simulink model "sim_pid_genetic"  (R2016b)
settings: Solver=ode5  StartTime=0.0  StopTime=10  FixedStep=0.01  RelTol=1e-3
values from neighbouring files (symbols this model uses):
  kd_ws = kd_val_dec(member,:)    [sim_genetic.m]
  ki_ws = ki_val_dec(member,:)    [sim_genetic.m]
  kp_ws = kp_val_dec(member,:)    [sim_genetic.m]
undefined symbols (not defined in the file or in its folder): DiscIntNeverNeededParam
settings Model: Creator=ismail.uzunlar  LastModifiedBy=Ismail

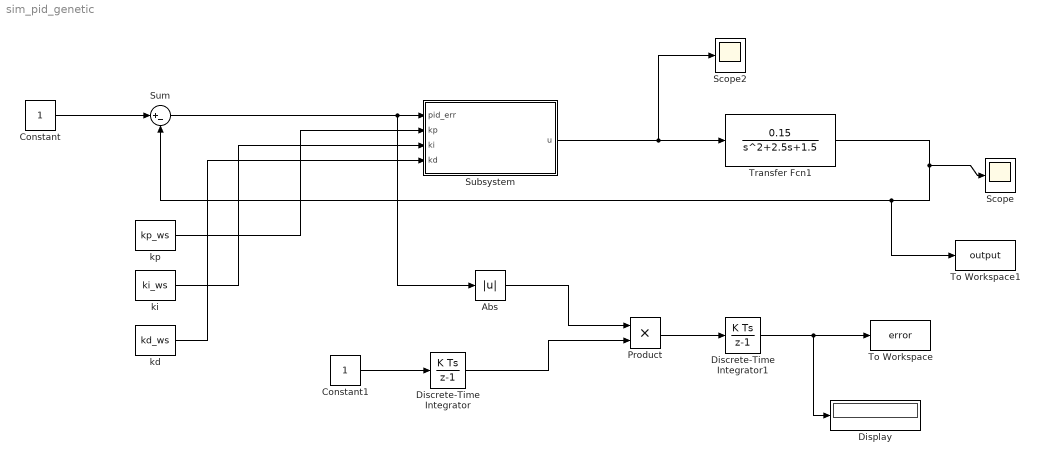
== system sim_pid_genetic ==
  Abs : Abs
  Constant : Constant
  Constant1 : Constant
  Discrete-Time Integrator : DiscreteIntegrator  gainval=1  InitialConditionSetting=State (most efficient)  SampleTime=-1  ICPrevOutput=DiscIntNeverNeededParam  ICPrevScaledInput=DiscIntNeverNeededParam
  Discrete-Time Integrator1 : DiscreteIntegrator  gainval=100  InitialConditionSetting=State (most efficient)  SampleTime=-1  ICPrevOutput=DiscIntNeverNeededParam  ICPrevScaledInput=DiscIntNeverNeededParam
  Display : Display
  Product : Product
  Scope : Scope
  Scope2 : Scope
  Subsystem : Subsystem
  Sum : Sum  Inputs=|+-
  To Workspace : ToWorkspace  VariableName=error  SaveFormat=Timeseries  SampleTime=-1
  To Workspace1 : ToWorkspace  VariableName=output  SaveFormat=Timeseries  SampleTime=-1
  Transfer Fcn1 : TransferFcn  Numerator=[0.15]  Denominator=[1 2.5 1.5]
  kd : Constant  Value=kd_ws
  ki : Constant  Value=ki_ws
  kp : Constant  Value=kp_ws
  wires:
  Subsystem/1(u) -> Scope2/1, Transfer Fcn1/1
  Constant/1 -> Sum/1
  Sum/1 -> Abs/1, Subsystem/1(pid_err)
  Transfer Fcn1/1 -> To Workspace1/1, Sum/2, Scope/1
  kp/1 -> Subsystem/2(kp)
  ki/1 -> Subsystem/3(ki)
  kd/1 -> Subsystem/4(kd)
  Constant1/1 -> Discrete-Time Integrator/1
  Discrete-Time Integrator/1 -> Product/2
  Abs/1 -> Product/1
  Product/1 -> Discrete-Time Integrator1/1
  Discrete-Time Integrator1/1 -> Display/1, To Workspace/1

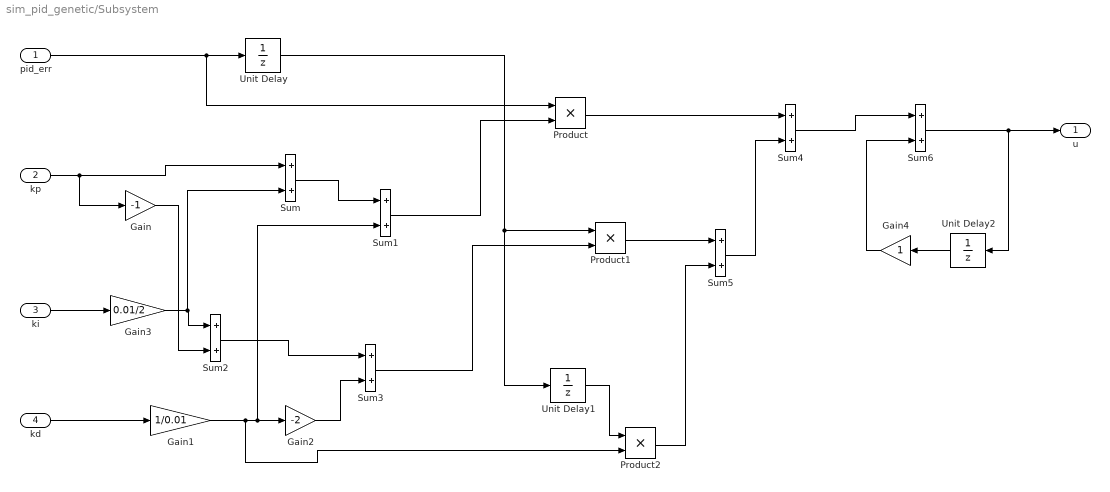
== system sim_pid_genetic/Subsystem ==
  pid_err : Inport
  kp : Inport  Port=2
  ki : Inport  Port=3
  kd : Inport  Port=4
  Gain : Gain  Gain=-1
  Gain1 : Gain  Gain=1/0.01
  Gain2 : Gain  Gain=-2
  Gain3 : Gain  Gain=0.01/2
  Gain4 : Gain
  Product : Product
  Product1 : Product
  Product2 : Product
  Sum{,1..6} (7 alike) : Sum
  Unit Delay : UnitDelay  SampleTime=-1
  Unit Delay1 : UnitDelay  SampleTime=-1
  Unit Delay2 : UnitDelay  SampleTime=-1
  u : Outport
  wires:
  pid_err/1 -> Product/1, Unit Delay/1
  kp/1 -> Sum/1, Gain/1
  Unit Delay1/1 -> Product2/1
  Unit Delay/1 -> Unit Delay1/1, Product1/1
  kd/1 -> Gain1/1
  Product1/1 -> Sum5/1
  Sum/1 -> Sum1/1
  Gain1/1 -> Product2/2, Sum1/2, Gain2/1
  Gain2/1 -> Sum3/2
  Gain/1 -> Sum2/2
  Sum4/1 -> Sum6/1
  Sum2/1 -> Sum3/1
  ki/1 -> Gain3/1
  Gain3/1 -> Sum/2, Sum2/1
  Product/1 -> Sum4/1
  Product2/1 -> Sum5/2
  Sum1/1 -> Product/2
  Sum5/1 -> Sum4/2
  Sum3/1 -> Product1/2
  Sum6/1 -> u/1, Unit Delay2/1
  Unit Delay2/1 -> Gain4/1
  Gain4/1 -> Sum6/2
